simulink model "problem_3_5"  (R2018a)
settings: Solver=FixedStepDiscrete  StartTime=0.0  StopTime=5e-3  FixedStep=Ts  RelTol=1e-3
InitFcn:
  | clc;clear;close all;
  | 
  | ms = 1e-3;
  | kHz = 1e3;
  | 
  | Ts = 0.01 * ms;
  | Fs = 1/Ts;
  | F1 = 10 * kHz;
  | F2 = 5  * kHz;
  | T = 0.5 * ms;
StopFcn:
  | n = 0:length(simout)-1;
  | w = [0:500]*pi/500;
  | X = dtft(simout,n,w);
  | magX = abs(X);
  | magX = magX / max(magX);
  | plot(w/pi,magX)
  | grid on;
  | title('DTFT Magnitude of FSK:  F1 = 10 kHz, F2 = 5 kHz, Tstop = 1 ms')
  | xlabel('digital frequency \omega  normalized by \pi')
  | ylabel('|X(e^{j\omega}|');
settings Model: Creator=Ryan  LastModifiedBy=Ryan

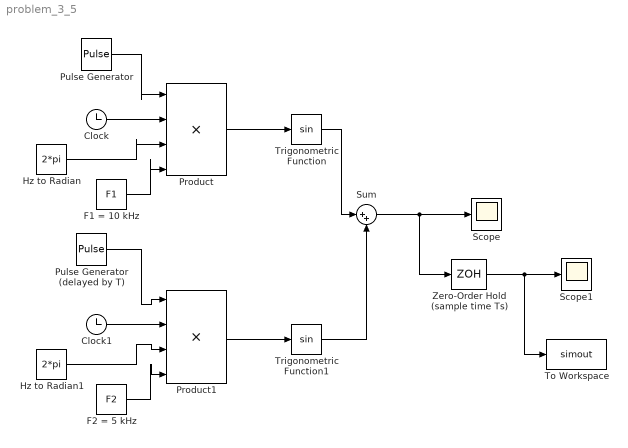
== system problem_3_5 ==
  Clock : Clock
  Clock1 : Clock
  F1 = 10 kHz : Constant  Value=F1
  F2 = 5 kHz : Constant  Value=F2
  Hz to Radian : Constant  Value=2*pi
  Hz to Radian1 : Constant  Value=2*pi
  Product : Product  Inputs=4
  Product1 : Product  Inputs=4
  Pulse Generator : DiscretePulseGenerator  PulseType=Time based  Period=2*T  PulseWidth=50
  Pulse Generator (delayed by T) : DiscretePulseGenerator  PulseType=Time based  Period=2*T  PulseWidth=50  PhaseDelay=T
  Scope : Scope
  Scope1 : Scope
  Sum : Sum  Inputs=|++
  To Workspace : ToWorkspace  VariableName=simout  SampleTime=-1
  Trigonometric Function : Trigonometry
  Trigonometric Function1 : Trigonometry
  Zero-Order Hold (sample time Ts) : ZeroOrderHold  SampleTime=Ts
  wires:
  Pulse Generator/1 -> Product/1
  Clock/1 -> Product/2
  Hz to Radian/1 -> Product/3
  F1 = 10 kHz/1 -> Product/4
  Clock1/1 -> Product1/2
  Pulse Generator (delayed by T)/1 -> Product1/1
  F2 = 5 kHz/1 -> Product1/4
  Hz to Radian1/1 -> Product1/3
  Product/1 -> Trigonometric Function/1
  Product1/1 -> Trigonometric Function1/1
  Trigonometric Function1/1 -> Sum/2
  Trigonometric Function/1 -> Sum/1
  Sum/1 -> Zero-Order Hold (sample time Ts)/1, Scope/1
  Zero-Order Hold (sample time Ts)/1 -> To Workspace/1, Scope1/1
